simulink model "MPC_HW2_Plant_Simulink"  (R2023b)
settings: Solver=ode4  StartTime=0.0  StopTime=20  FixedStep=1e-3  RelTol=1e-3
values from neighbouring files (symbols this model uses):
  V_ref = 60 /3.6    (= 16.6666666667)    [veh_parameters.m]
undefined symbols (not defined in the file or in its folder): controller_choice, data, init, input, par, Ts
libraries: simulink x6
settings Model: Creator=bshyrokau  LastModifiedBy=india
settings SolverCC: AlgebraicLoopSolver=TrustRegion
settings DataIOCC: SaveOutput=off  SignalLogging=off  DSMLogging=off  SaveTime=off  ReturnWorkspaceOutputs=off
settings OptimizationCC: ReuseModelBlockBuffer=off  LifeSpan=inf
settings DebuggingCC: UnconnectedInputMsg=warning  UnconnectedOutputMsg=warning  UnconnectedLineMsg=warning  AllowSymbolicDim=off  SFUnexpectedBacktrackingDiag=warning  SFNoUnconditionalDefaultTransitionDiag=warning  SFExecutionAtInitializationDiag=none  ArithmeticOperatorsInVariantConditions=warning
settings ModelReferenceCC: EnableRefExpFcnMdlSchedulingChecks=on  PropagateSignalLabelsOutOfModel=off
settings SFSimCC: SimUseLocalCustomCode=off  CustomCodeUndefinedFunction=UseInterfaceOnly
settings RTWCC: RTWUseLocalCustomCode=off  DLArmComputeVersion=19.05
settings CodeAppCC: StateflowObjectComments=on
settings GRTTargetCC: TargetLangStandard=C89/C90 (ANSI)
settings ConfigComp: CovMetricSettings=dw  CovSaveCumulativeToWorkspaceVar=on  CovSaveSingleToWorkspaceVar=on  CovExternalEMLEnable=off
settings SimscapeCC: SimscapeNormalizeSystem=off
settings ConfigurationSet: Description=SimMechanics 2G

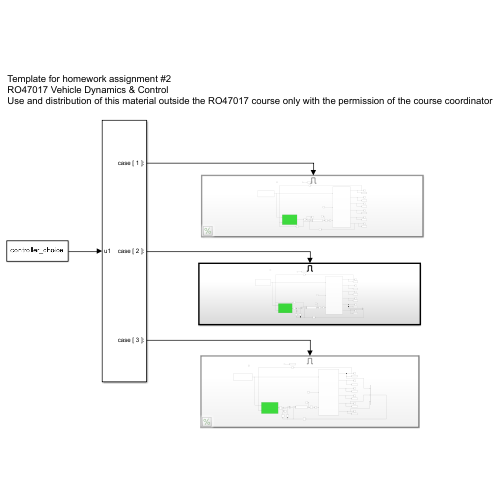
[thumbnail: Simulink's stored preview of the top-level diagram]
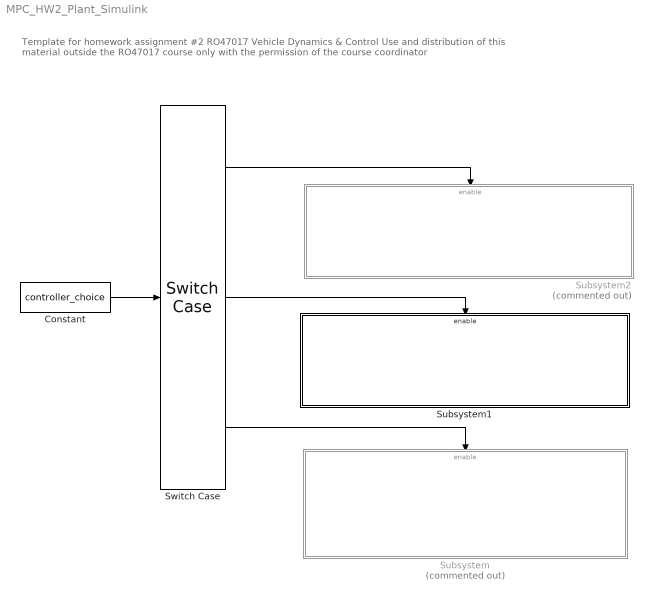
== system MPC_HW2_Plant_Simulink ==
  note: Template for homework assignment #2
      | RO47017 Vehicle Dynamics & Control
      | Use and distribution of this material outside the RO47017 course only with the permission of the course coordinator
  Constant : Constant  Value=controller_choice
  Subsystem : Subsystem  Commented=on
  Subsystem1 : Subsystem
  Subsystem2 : Subsystem  Commented=on
  Switch Case : SwitchCase  CaseConditions={1 2 3}  ShowDefaultCase=off
  wires:
  Switch Case/2 -> Subsystem1/Enable
  Switch Case/3 -> Subsystem/Enable
  Constant/1 -> Switch Case/1
  Switch Case/1 -> Subsystem2/Enable

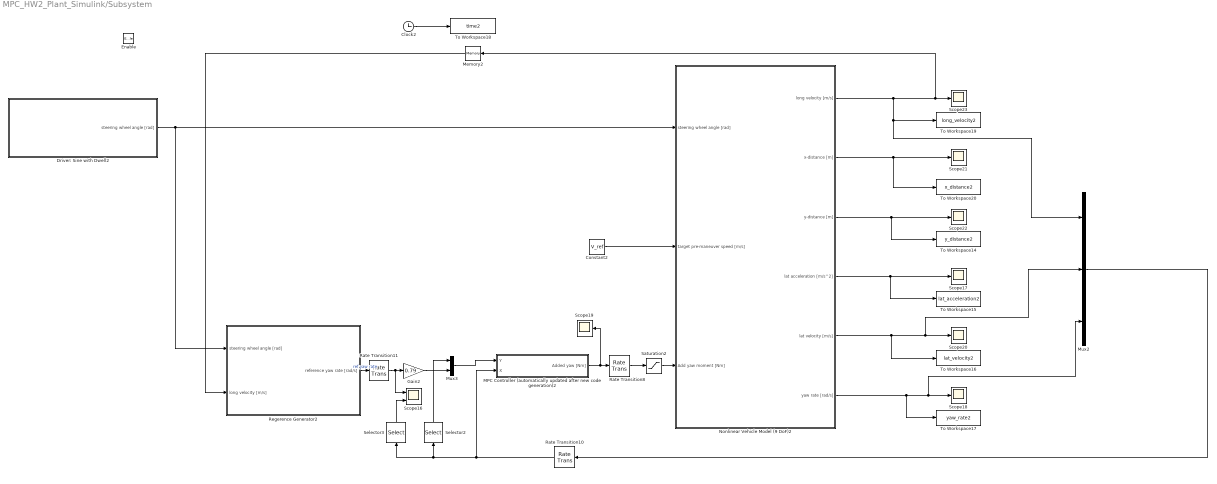
== system MPC_HW2_Plant_Simulink/Subsystem ==
  Enable : EnablePort
  Clock2 : Clock
  Constant2 : Constant  Value=V_ref
  Driver: Sine with Dwell2 : Subsystem
  Gain2 : Gain  Gain=0.79
  MPC Controller (automatically updated after new code generation)2 : Subsystem
  Memory2 : Memory  InitialCondition=V_ref
  Mux2 : Mux  Inputs=3
  Mux3 : Mux  Inputs=2
  Nonlinear Vehicle Model (9 DoF)2 : Subsystem
      mask help: Simulink:masks:GenSFuncDesc_MD
      mask Help: eval('feval(''rtwprivate'',''rtwhelpview'',''rtw_sfcn_block'')');
  Rate Transition10 : RateTransition  InitialCondition=[V_ref 0 0]  OutPortSampleTime=Ts
  Rate Transition11 : RateTransition  OutPortSampleTime=Ts
  Rate Transition8 : RateTransition
  Regerence Generator2 : Subsystem
  Saturation2 : Saturate  UpperLimit=10000  LowerLimit=-10000
  Scope16 : Scope  NumInputPorts=2
  Scope{17..23} (7 alike) : Scope
  Selector2 : Selector  InputPortWidth=3  IndexOptions=Index vector (dialog)  Indices=[1 2]  OutputSizes=1
  Selector3 : Selector  InputPortWidth=3  IndexOptions=Index vector (dialog)  Indices=3  OutputSizes=1
  To Workspace14 : ToWorkspace  VariableName=y_distance2  SampleTime=-1
  To Workspace15 : ToWorkspace  VariableName=lat_acceleration2  SampleTime=-1
  To Workspace16 : ToWorkspace  VariableName=lat_velocity2  SampleTime=-1
  To Workspace17 : ToWorkspace  VariableName=yaw_rate2  SampleTime=-1
  To Workspace18 : ToWorkspace  VariableName=time2  SampleTime=-1
  To Workspace19 : ToWorkspace  VariableName=long_velocity2  SampleTime=-1
  To Workspace20 : ToWorkspace  VariableName=x_distance2  SampleTime=-1
  wires:
  Nonlinear Vehicle Model (9 DoF)2/6(yaw rate [rad/s]) -> Mux2/3, Scope18/1, To Workspace17/1
  Rate Transition10/1 -> Selector3/1, Selector2/1, MPC Controller (automatically updated after new code generation)2/2(X)
  Driver: Sine with Dwell2/1(steering wheel angle [rad]) -> Regerence Generator2/1(steering wheel angle [rad]), Nonlinear Vehicle Model (9 DoF)2/1(steering wheel angle [rad])
  Nonlinear Vehicle Model (9 DoF)2/1(long velocity [m/s]) -> Mux2/1, To Workspace19/1, Memory2/1, Scope23/1
  Nonlinear Vehicle Model (9 DoF)2/5(lat velocity [m/s]) -> To Workspace16/1, Mux2/2, Scope20/1
  Nonlinear Vehicle Model (9 DoF)2/2(x-distance [m]) -> To Workspace20/1, Scope21/1
  Nonlinear Vehicle Model (9 DoF)2/4(lat acceleration [m/s^2]) -> To Workspace15/1, Scope17/1
  MPC Controller (automatically updated after new code generation)2/1(Added yaw [Nm]) -> Scope19/1, Rate Transition8/1
  Mux3/1 -> MPC Controller (automatically updated after new code generation)2/1(Y)
  Mux2/1 -> Rate Transition10/1
  Nonlinear Vehicle Model (9 DoF)2/3(y-distance [m]) -> To Workspace14/1, Scope22/1
  Memory2/1 -> Regerence Generator2/2(long velocity [m/s])
  Selector3/1 -> Scope16/2
  Regerence Generator2/1(reference yaw rate [rad/s]) -> Rate Transition11/1  "ref yaw rate"
  Rate Transition11/1 -> Scope16/1, Gain2/1
  Saturation2/1 -> Nonlinear Vehicle Model (9 DoF)2/3(Add yaw moment [Nm])
  Clock2/1 -> To Workspace18/1
  Rate Transition8/1 -> Saturation2/1
  Constant2/1 -> Nonlinear Vehicle Model (9 DoF)2/2(target pre-maneuver speed [m/s])
  Gain2/1 -> Mux3/2
  Selector2/1 -> Mux3/1

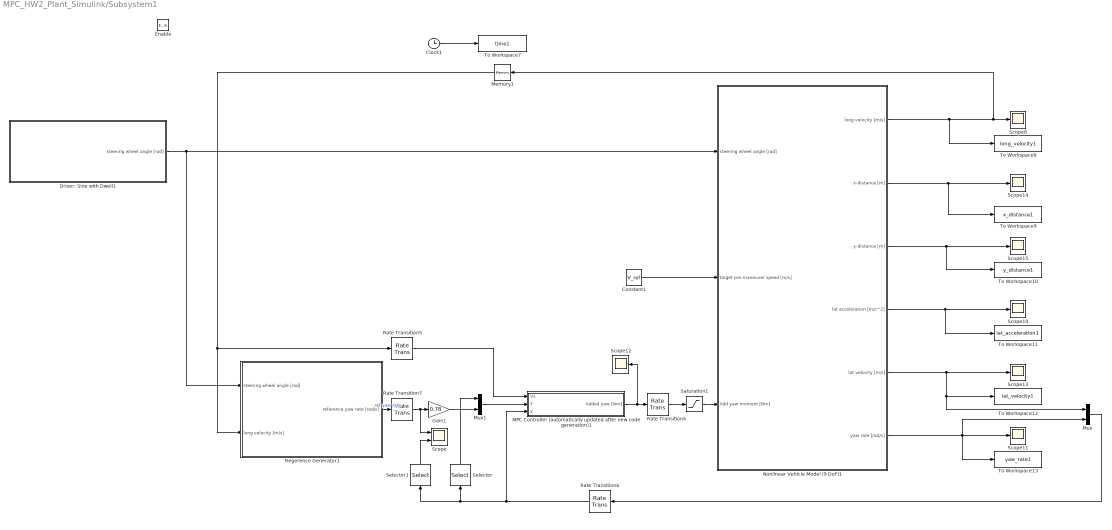
== system MPC_HW2_Plant_Simulink/Subsystem1 ==
  Enable : EnablePort
  Clock1 : Clock
  Constant1 : Constant  Value=V_ref
  Driver: Sine with Dwell1 : Subsystem
  Gain1 : Gain  Gain=0.78
  MPC Controller (automatically updated after new code generation)1 : Subsystem
  Memory1 : Memory  InitialCondition=V_ref
  Mux : Mux  Inputs=2
  Mux1 : Mux  Inputs=2
  Nonlinear Vehicle Model (9 DoF)1 : Subsystem
      mask help: Simulink:masks:GenSFuncDesc_MD
      mask Help: eval('feval(''rtwprivate'',''rtwhelpview'',''rtw_sfcn_block'')');
  Rate Transition4 : RateTransition
  Rate Transition5 : RateTransition  InitialCondition=V_ref  OutPortSampleTime=Ts
  Rate Transition6 : RateTransition  InitialCondition=[0 0]  OutPortSampleTime=Ts
  Rate Transition7 : RateTransition  OutPortSampleTime=Ts
  Regerence Generator1 : Subsystem
  Saturation1 : Saturate  UpperLimit=10000  LowerLimit=-10000
  Scope : Scope  NumInputPorts=2
  Scope{8,10..15} (7 alike) : Scope
  Selector : Selector  InputPortWidth=2  IndexOptions=Index vector (dialog)  Indices=1  OutputSizes=1
  Selector1 : Selector  InputPortWidth=2  IndexOptions=Index vector (dialog)  Indices=2  OutputSizes=1
  To Workspace10 : ToWorkspace  VariableName=y_distance1  SampleTime=-1
  To Workspace11 : ToWorkspace  VariableName=lat_acceleration1  SampleTime=-1
  To Workspace12 : ToWorkspace  VariableName=lat_velocity1  SampleTime=-1
  To Workspace13 : ToWorkspace  VariableName=yaw_rate1  SampleTime=-1
  To Workspace7 : ToWorkspace  VariableName=time1  SampleTime=-1
  To Workspace8 : ToWorkspace  VariableName=long_velocity1  SampleTime=-1
  To Workspace9 : ToWorkspace  VariableName=x_distance1  SampleTime=-1
  wires:
  Rate Transition4/1 -> Saturation1/1
  Nonlinear Vehicle Model (9 DoF)1/3(y-distance [m]) -> To Workspace10/1, Scope15/1
  MPC Controller (automatically updated after new code generation)1/1(Added yaw [Nm]) -> Scope12/1, Rate Transition4/1
  Constant1/1 -> Nonlinear Vehicle Model (9 DoF)1/2(target pre-maneuver speed [m/s])
  Rate Transition6/1 -> Selector1/1, Selector/1, MPC Controller (automatically updated after new code generation)1/3(X)
  Rate Transition5/1 -> MPC Controller (automatically updated after new code generation)1/1(Vx)
  Nonlinear Vehicle Model (9 DoF)1/2(x-distance [m]) -> To Workspace9/1, Scope14/1
  Mux/1 -> Rate Transition6/1
  Saturation1/1 -> Nonlinear Vehicle Model (9 DoF)1/3(Add yaw moment [Nm])
  Nonlinear Vehicle Model (9 DoF)1/1(long velocity [m/s]) -> To Workspace8/1, Memory1/1, Scope8/1
  Regerence Generator1/1(reference yaw rate [rad/s]) -> Rate Transition7/1  "ref yaw rate"
  Memory1/1 -> Regerence Generator1/2(long velocity [m/s]), Rate Transition5/1
  Driver: Sine with Dwell1/1(steering wheel angle [rad]) -> Regerence Generator1/1(steering wheel angle [rad]), Nonlinear Vehicle Model (9 DoF)1/1(steering wheel angle [rad])
  Nonlinear Vehicle Model (9 DoF)1/6(yaw rate [rad/s]) -> Mux/2, Scope11/1, To Workspace13/1
  Clock1/1 -> To Workspace7/1
  Nonlinear Vehicle Model (9 DoF)1/4(lat acceleration [m/s^2]) -> To Workspace11/1, Scope10/1
  Nonlinear Vehicle Model (9 DoF)1/5(lat velocity [m/s]) -> Mux/1, To Workspace12/1, Scope13/1
  Mux1/1 -> MPC Controller (automatically updated after new code generation)1/2(Y)
  Selector1/1 -> Scope/2
  Gain1/1 -> Mux1/2
  Rate Transition7/1 -> Scope/1, Gain1/1
  Selector/1 -> Mux1/1

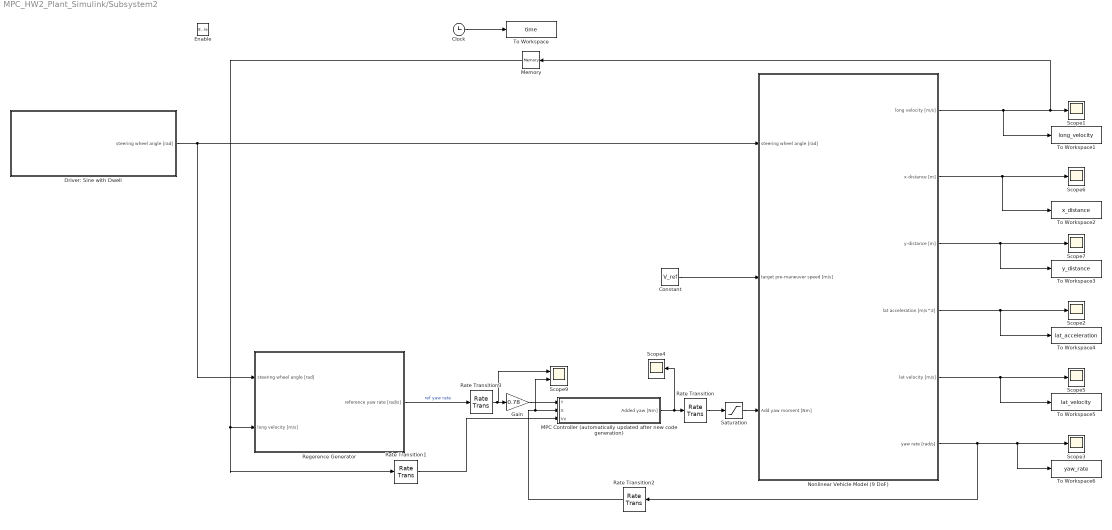
== system MPC_HW2_Plant_Simulink/Subsystem2 ==
  Enable : EnablePort
  Clock : Clock
  Constant : Constant  Value=V_ref
  Driver: Sine with Dwell : Subsystem
  Gain : Gain  Gain=0.78
  MPC Controller (automatically updated after new code generation) : Subsystem
  Memory : Memory  InitialCondition=V_ref
  Nonlinear Vehicle Model (9 DoF) : Subsystem
      mask help: Simulink:masks:GenSFuncDesc_MD
      mask Help: eval('feval(''rtwprivate'',''rtwhelpview'',''rtw_sfcn_block'')');
  Rate Transition : RateTransition
  Rate Transition1 : RateTransition  InitialCondition=V_ref  OutPortSampleTime=Ts
  Rate Transition2 : RateTransition  OutPortSampleTime=Ts
  Rate Transition3 : RateTransition  OutPortSampleTime=Ts
  Regerence Generator : Subsystem
  Saturation : Saturate  UpperLimit=10000  LowerLimit=-10000
  Scope{1..7} (7 alike) : Scope
  Scope9 : Scope  NumInputPorts=2
  To Workspace : ToWorkspace  VariableName=time  SampleTime=-1
  To Workspace1 : ToWorkspace  VariableName=long_velocity  SampleTime=-1
  To Workspace2 : ToWorkspace  VariableName=x_distance  SampleTime=-1
  To Workspace3 : ToWorkspace  VariableName=y_distance  SampleTime=-1
  To Workspace4 : ToWorkspace  VariableName=lat_acceleration  SampleTime=-1
  To Workspace5 : ToWorkspace  VariableName=lat_velocity  SampleTime=-1
  To Workspace6 : ToWorkspace  VariableName=yaw_rate  SampleTime=-1
  wires:
  Driver: Sine with Dwell/1(steering wheel angle [rad]) -> Regerence Generator/1(steering wheel angle [rad]), Nonlinear Vehicle Model (9 DoF)/1(steering wheel angle [rad])
  Nonlinear Vehicle Model (9 DoF)/6(yaw rate [rad/s]) -> Rate Transition2/1, Scope3/1, To Workspace6/1
  Nonlinear Vehicle Model (9 DoF)/3(y-distance [m]) -> To Workspace3/1, Scope7/1
  Nonlinear Vehicle Model (9 DoF)/2(x-distance [m]) -> To Workspace2/1, Scope6/1
  Nonlinear Vehicle Model (9 DoF)/1(long velocity [m/s]) -> To Workspace1/1, Memory/1, Scope1/1
  MPC Controller (automatically updated after new code generation)/1(Added yaw [Nm]) -> Scope4/1, Rate Transition/1
  Gain/1 -> MPC Controller (automatically updated after new code generation)/1(Y)
  Nonlinear Vehicle Model (9 DoF)/5(lat velocity [m/s]) -> To Workspace5/1, Scope5/1
  Rate Transition2/1 -> Scope9/2, MPC Controller (automatically updated after new code generation)/2(X)
  Nonlinear Vehicle Model (9 DoF)/4(lat acceleration [m/s^2]) -> To Workspace4/1, Scope2/1
  Constant/1 -> Nonlinear Vehicle Model (9 DoF)/2(target pre-maneuver speed [m/s])
  Rate Transition3/1 -> Scope9/1, Gain/1
  Memory/1 -> Rate Transition1/1, Regerence Generator/2(long velocity [m/s])
  Clock/1 -> To Workspace/1
  Rate Transition1/1 -> MPC Controller (automatically updated after new code generation)/3(Vx)
  Saturation/1 -> Nonlinear Vehicle Model (9 DoF)/3(Add yaw moment [Nm])
  Regerence Generator/1(reference yaw rate [rad/s]) -> Rate Transition3/1  "ref yaw rate"
  Rate Transition/1 -> Saturation/1

== system MPC_HW2_Plant_Simulink/Subsystem/Driver: Sine with Dwell2 ==
  Constant1 : Constant
  Lookup Table1 : Lookup  InputValues=[0:0.1:3*pi/2 3*pi/2+eps]*0.7  Table=sin([0:0.1:3*pi/2 3*pi/2+eps])  LookUpMeth=Interpolation-Use End Values  SaturateOnIntegerOverflow=off
  Lookup Table2 : Lookup  InputValues=[3*pi/2:0.1:2*pi 2*pi+eps]*0.7  Table=sin([3*pi/2:0.1:2*pi 2*pi+eps])  LookUpMeth=Interpolation-Use End Values  SaturateOnIntegerOverflow=off
  Ramp6 : simulink/Sources/Ramp  slope=pi  start=10  InitialOutput=0
  Ramp7 : simulink/Sources/Ramp  slope=pi  start=10+0.5  InitialOutput=0
  Subtract1 : Sum  Inputs=+++
  amplitude : Gain  Gain=120
  deg2rad : Gain  Gain=pi / 180
  steering wheel angle [rad] : Outport  VectorParamsAs1DForOutWhenUnconnected=off
  wires:
  Ramp6/1 -> Lookup Table1/1
  Ramp7/1 -> Lookup Table2/1
  Lookup Table2/1 -> Subtract1/2
  Lookup Table1/1 -> Subtract1/1
  Constant1/1 -> Subtract1/3
  Subtract1/1 -> amplitude/1
  amplitude/1 -> deg2rad/1
  deg2rad/1 -> steering wheel angle [rad]/1

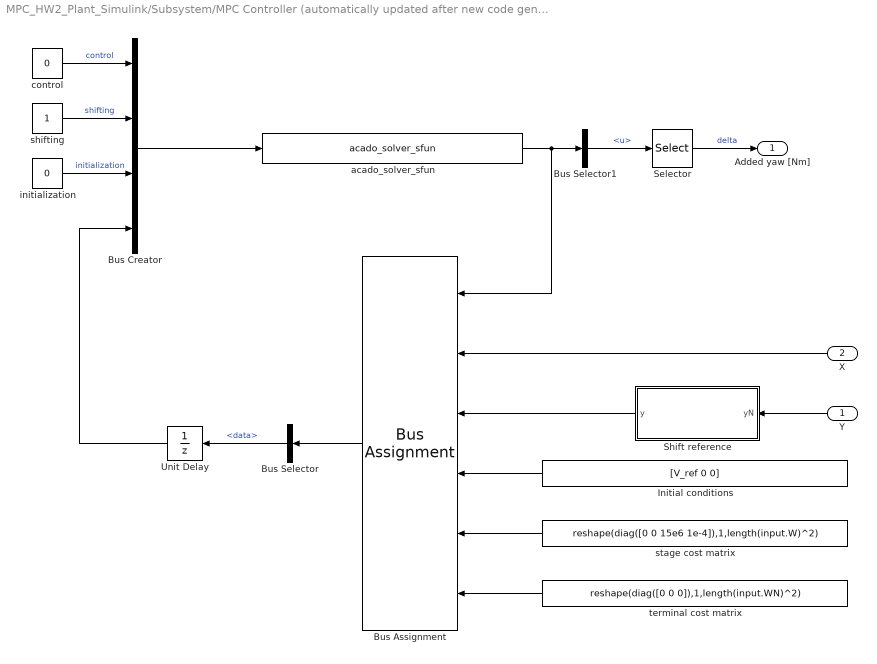
== system MPC_HW2_Plant_Simulink/Subsystem/MPC Controller (automatically updated after new code generation)2 ==
  Y : Inport
  X : Inport  Port=2
  Bus Assignment : BusAssignment  AssignedSignals=data.x0,data.y,data.yN,data.W,data.WN
  Bus Creator : BusCreator  Inputs=4  OutDataTypeStr=Bus: ACADOinput
  Bus Selector : BusSelector  OutputSignals=data
  Bus Selector1 : BusSelector  OutputSignals=data.u
  Initial conditions : Constant  Value=[V_ref 0 0]
  Selector : Selector  InputPortWidth=Np  IndexOptions=Starting index (dialog)  Indices=[1]  OutputSizes=1
  Shift reference : MATLAB Function  TreatAsAtomicUnit=on
  Unit Delay : UnitDelay  InitialCondition=init  SampleTime=Ts  HasFrameUpgradeWarning=on
  acado_solver_sfun : S-Function  FunctionName=acado_solver_sfun  SFunctionDeploymentMode=off  EnableBusSupport=off  mask(Legacy Function){SFunctionSpec=acado_step(ACADOinput u1[1], ACADOoutput y1[1]), ShowSpec=on}
      mask prompts: ShowSpec "Display function specification"
      mask help:
      | This block allows you to call the legacy functions specified by the following Legacy Code Tool definition:
      | def.SFunctionName = 'acado_solver_sfun';
      | def.OutputFcnSpec = 'acado_step(ACADOinput u1[1], ACADOoutput y1[1])';
      | def.StartFcnSpec = 'acado_initialize( void )';
      | def.TerminateFcnSpec = 'acado_cleanup( void )';
      | def.HeaderFiles = {'acado_common.h', 'acado_solver_sfunction.h'};
      | def.SourceFiles = {'acado_solver.c', 'acado_integrator.c', 'acado_auxiliary_functions.c', 'acado_solver_sfunction.c', 'acado_qpoases3_interface.c', 'qpoases3\src\Bounds.c', 'qpoases3\src\Constraints.c', 'qpoases3\src\Indexlist.c', 'qpoases3\src\Matrices.c', 'qpoases3\src\MessageHandling.c', 'qpoases3\src\Options.c', 'qpoases3\src\Flipper.c', 'qpoases3\src\QProblem.c', 'qpoases3\src\QProblemB.c', 'qpoases3\src\Utils.c'};
      mask Help: <p>This block was generated automatically by the Legacy Code Tool. For detailed help on this tool, call<a href="matlab:legacy_code('help')"> legacy_code('help')</a>.</p>
      mask Callback ShowSpec:
      | if strcmp(get_param(gcbh, 'ShowSpec'), 'on')
      |   set_param(gcbh, 'MaskDisplay', sprintf('fprintf(''%s'');', get_param(gcbh, 'SFunctionSpec')));
      | else
      |   set_param(gcbh, 'MaskDisplay', sprintf('fprintf(''%s'');', get_param(gcbh, 'FunctionName')));
      | end
      mask Display: fprintf('acado_step(ACADOinput u1[1], ACADOoutput y1[1])');
  control : Constant  Value=0  OutDataTypeStr=int32
  initialization : Constant  Value=0  OutDataTypeStr=int32
  shifting : Constant  OutDataTypeStr=int32
  stage cost matrix : Constant  Value=reshape(diag([0 0 15e6 1e-4]),1,length(input.W)^2)
  terminal cost matrix : Constant  Value=reshape(diag([0 0 0]),1,length(input.WN)^2)
  Added yaw [Nm] : Outport
  wires:
  control/1 -> Bus Creator/1  "control"
  Bus Selector1/1 -> Selector/1  "<u>"
  initialization/1 -> Bus Creator/3  "initialization"
  acado_solver_sfun/1 -> Bus Selector1/1, Bus Assignment/1
  shifting/1 -> Bus Creator/2  "shifting"
  Bus Assignment/1 -> Bus Selector/1
  terminal cost matrix/1 -> Bus Assignment/6
  Initial conditions/1 -> Bus Assignment/4
  Shift reference/1(y) -> Bus Assignment/3
  stage cost matrix/1 -> Bus Assignment/5
  Bus Selector/1 -> Unit Delay/1  "<data>"
  Unit Delay/1 -> Bus Creator/4
  Bus Creator/1 -> acado_solver_sfun/1
  Selector/1 -> Added yaw [Nm]/1  "delta"
  Y/1 -> Shift reference/1(yN)
  X/1 -> Bus Assignment/2

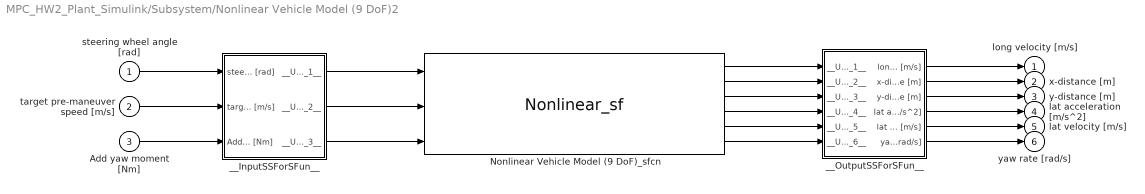
== system MPC_HW2_Plant_Simulink/Subsystem/Nonlinear Vehicle Model (9 DoF)2 ==
  steering wheel angle [rad] : Inport
  target pre-maneuver speed [m/s] : Inport  Port=2
  Add yaw moment [Nm] : Inport  Port=3
  Nonlinear Vehicle Model (9 DoF)_sfcn : S-Function  FunctionName=Nonlinear_sf  SFunctionModules=""  SFunctionDeploymentMode=off  EnableBusSupport=off  mask{rtw_sf_name=Nonlinear_sf, showVar=off}
      mask prompts: rtw_sf_name "Simulink:masks:GenSFuncName_MP"; showVar "Simulink:masks:GenSFuncShowModuleList_MP"
      mask help: Simulink:masks:GenSFuncDesc_MD
      mask init:
      | displist = '';
      | if ~strcmp(get_param(gcb, 'FunctionName'), rtw_sf_name);
      |   set_param(gcb, 'FunctionName', rtw_sf_name);
      | end
      | % Check if we are generating code
      | rtw_mode = false;
      | if strcmpi(get_param(bdroot(gcb),'SimulationStatus'),'Initializing')
      | 	rtw_mode = strcmpi(get_param(bdroot(gcb),'BuildingRTWCode'),'on') && ...
      | 		~strcmpi(get_param(bdroot(gcb),'TargetStyle'),'SimulationTarget');
      | end
      | if showVar || rtw_mode
      | 	if exist('rtwsfunc') == 2 | exist('rtwsfunc') == 6
      | 		tmplist = rtwsfunc(rtw_sf_name,gcb);
      | 		tmplist = DAStudio.message('Simulink:masks:GenSFuncListOfModules_IC', tmplist);
      | 	elseif showVar
      | 		tmplist1 = DAStudio.message('Simulink:masks:GenSFuncListOfModules_IC', '');
      |         tmplist2 = DAStudio.message('Simulink:masks:GenSFuncNotLicensed_IC');
      |         tmplist = [tmplist1 tmplist2];
      |  	end
      | end
      | if showVar
      |   displist = tmplist;
      | end
      settings: CopyFcn=|
      | if ~strcmp(get_param(gcb,'Linkstatus'),'none') && ...
      | ~strcmp(get_param(gcb,'Linkstatus'),'implicit')
      |   set_param(gcb,'LinkStatus','none');
      | end
      mask Help: eval('feval(''rtwprivate'',''rtwhelpview'',''rtw_sfcn_block'')');
      mask Display:
      | port_label('input',1,'steering wheel angle [rad]');
      | port_label('input',2,'target pre-maneuver speed [m/s]');
      | port_label('input',3,'Add yaw moment [Nm]');
      | port_label('output',1,'long velocity [m/s]');
      | port_label('output',2,'x-distance [m]');
      | port_label('output',3,'y-distance [m]');
      | port_label('output',4,'lat acceleration [m/s^2]');
      | port_label('output',5,'lat velocity [m/s]');
      | port_label('output',6,'yaw rate [rad/s]');
  __InputSSForSFun__ : Subsystem
  __OutputSSForSFun__ : Subsystem
  long velocity [m/s] : Outport  VectorParamsAs1DForOutWhenUnconnected=off
  x-distance [m] : Outport  Port=2  VectorParamsAs1DForOutWhenUnconnected=off
  y-distance [m] : Outport  Port=3  VectorParamsAs1DForOutWhenUnconnected=off
  lat acceleration [m/s^2] : Outport  Port=4  VectorParamsAs1DForOutWhenUnconnected=off
  lat velocity [m/s] : Outport  Port=5  VectorParamsAs1DForOutWhenUnconnected=off
  yaw rate [rad/s] : Outport  Port=6  VectorParamsAs1DForOutWhenUnconnected=off
  wires:
  steering wheel angle [rad]/1 -> __InputSSForSFun__/1(steering wheel angle [rad])
  target pre-maneuver speed [m/s]/1 -> __InputSSForSFun__/2(target pre-maneuver speed [m/s])
  __InputSSForSFun__/1(__UniqueOutportName__1__) -> Nonlinear Vehicle Model (9 DoF)_sfcn/1
  __InputSSForSFun__/3(__UniqueOutportName__3__) -> Nonlinear Vehicle Model (9 DoF)_sfcn/3
  Nonlinear Vehicle Model (9 DoF)_sfcn/1 -> __OutputSSForSFun__/1(__UniqueInportName__1__)
  Nonlinear Vehicle Model (9 DoF)_sfcn/2 -> __OutputSSForSFun__/2(__UniqueInportName__2__)
  Nonlinear Vehicle Model (9 DoF)_sfcn/3 -> __OutputSSForSFun__/3(__UniqueInportName__3__)
  Nonlinear Vehicle Model (9 DoF)_sfcn/4 -> __OutputSSForSFun__/4(__UniqueInportName__4__)
  Nonlinear Vehicle Model (9 DoF)_sfcn/5 -> __OutputSSForSFun__/5(__UniqueInportName__5__)
  Nonlinear Vehicle Model (9 DoF)_sfcn/6 -> __OutputSSForSFun__/6(__UniqueInportName__6__)
  __OutputSSForSFun__/1(long velocity [m/s]) -> long velocity [m/s]/1
  __OutputSSForSFun__/2(x-distance [m]) -> x-distance [m]/1
  __OutputSSForSFun__/3(y-distance [m]) -> y-distance [m]/1
  __OutputSSForSFun__/4(lat acceleration [m/s^2]) -> lat acceleration [m/s^2]/1
  __OutputSSForSFun__/5(lat velocity [m/s]) -> lat velocity [m/s]/1
  __OutputSSForSFun__/6(yaw rate [rad/s]) -> yaw rate [rad/s]/1
  __InputSSForSFun__/2(__UniqueOutportName__2__) -> Nonlinear Vehicle Model (9 DoF)_sfcn/2
  Add yaw moment [Nm]/1 -> __InputSSForSFun__/3(Add yaw moment [Nm])

== system MPC_HW2_Plant_Simulink/Subsystem/Regerence Generator2 ==
  note: yawr_ref
  note: nonlinear response
  note: delta
  note: u
  steering wheel angle [rad] : Inport
  long velocity [m/s] : Inport  Port=2
  MATLAB Function : MATLAB Function  TreatAsAtomicUnit=on
  MATLAB Function1 : MATLAB Function  TreatAsAtomicUnit=on
  Transfer Fcn : TransferFcn  Numerator=[par.wn^2*par.tau par.wn^2]  Denominator=[1 2*par.kseta*par.wn par.wn^2]
  steering ratio : Gain  Gain=1/ par.i_steer
  reference yaw rate [rad/s] : Outport  VectorParamsAs1DForOutWhenUnconnected=off
  wires:
  steering wheel angle [rad]/1 -> steering ratio/1
  steering ratio/1 -> MATLAB Function/1(delta)
  long velocity [m/s]/1 -> MATLAB Function1/2(u), MATLAB Function/2(u)
  MATLAB Function/1(yawr_ss) -> MATLAB Function1/1(yawr_ss)
  MATLAB Function1/1(yawr_sat) -> Transfer Fcn/1
  Transfer Fcn/1 -> reference yaw rate [rad/s]/1

== system MPC_HW2_Plant_Simulink/Subsystem1/Driver: Sine with Dwell1 ==
  Constant1 : Constant
  Lookup Table1 : Lookup  InputValues=[0:0.1:3*pi/2 3*pi/2+eps]*0.7  Table=sin([0:0.1:3*pi/2 3*pi/2+eps])  LookUpMeth=Interpolation-Use End Values  SaturateOnIntegerOverflow=off
  Lookup Table2 : Lookup  InputValues=[3*pi/2:0.1:2*pi 2*pi+eps]*0.7  Table=sin([3*pi/2:0.1:2*pi 2*pi+eps])  LookUpMeth=Interpolation-Use End Values  SaturateOnIntegerOverflow=off
  Ramp6 : simulink/Sources/Ramp  slope=pi  start=10  InitialOutput=0
  Ramp7 : simulink/Sources/Ramp  slope=pi  start=10+0.5  InitialOutput=0
  Subtract1 : Sum  Inputs=+++
  amplitude : Gain  Gain=120
  deg2rad : Gain  Gain=pi / 180
  steering wheel angle [rad] : Outport  VectorParamsAs1DForOutWhenUnconnected=off
  wires:
  Ramp6/1 -> Lookup Table1/1
  Ramp7/1 -> Lookup Table2/1
  Lookup Table2/1 -> Subtract1/2
  Lookup Table1/1 -> Subtract1/1
  Constant1/1 -> Subtract1/3
  Subtract1/1 -> amplitude/1
  amplitude/1 -> deg2rad/1
  deg2rad/1 -> steering wheel angle [rad]/1

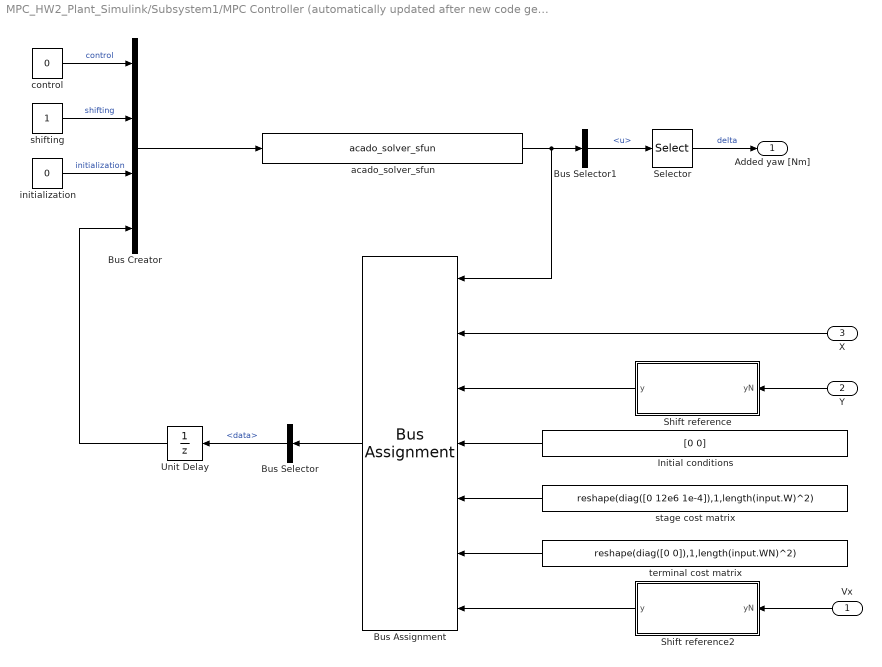
== system MPC_HW2_Plant_Simulink/Subsystem1/MPC Controller (automatically updated after new code generation)1 ==
  Vx : Inport
  Y : Inport  Port=2
  X : Inport  Port=3
  Bus Assignment : BusAssignment  AssignedSignals=data.x0,data.y,data.yN,data.W,data.WN,data.od
  Bus Creator : BusCreator  Inputs=4  OutDataTypeStr=Bus: ACADOinput
  Bus Selector : BusSelector  OutputSignals=data
  Bus Selector1 : BusSelector  OutputSignals=data.u
  Initial conditions : Constant  Value=[0 0]
  Selector : Selector  InputPortWidth=Np  IndexOptions=Starting index (dialog)  Indices=[1]  OutputSizes=1
  Shift reference : MATLAB Function  TreatAsAtomicUnit=on
  Shift reference2 : MATLAB Function  TreatAsAtomicUnit=on
  Unit Delay : UnitDelay  InitialCondition=init  SampleTime=Ts  HasFrameUpgradeWarning=on
  acado_solver_sfun : S-Function  FunctionName=acado_solver_sfun  SFunctionDeploymentMode=off  EnableBusSupport=off  mask(Legacy Function){SFunctionSpec=acado_step(ACADOinput u1[1], ACADOoutput y1[1]), ShowSpec=on}
      mask prompts: ShowSpec "Display function specification"
      mask help:
      | This block allows you to call the legacy functions specified by the following Legacy Code Tool definition:
      | def.SFunctionName = 'acado_solver_sfun';
      | def.OutputFcnSpec = 'acado_step(ACADOinput u1[1], ACADOoutput y1[1])';
      | def.StartFcnSpec = 'acado_initialize( void )';
      | def.TerminateFcnSpec = 'acado_cleanup( void )';
      | def.HeaderFiles = {'acado_common.h', 'acado_solver_sfunction.h'};
      | def.SourceFiles = {'acado_solver.c', 'acado_integrator.c', 'acado_auxiliary_functions.c', 'acado_solver_sfunction.c', 'acado_qpoases3_interface.c', 'qpoases3\src\Bounds.c', 'qpoases3\src\Constraints.c', 'qpoases3\src\Indexlist.c', 'qpoases3\src\Matrices.c', 'qpoases3\src\MessageHandling.c', 'qpoases3\src\Options.c', 'qpoases3\src\Flipper.c', 'qpoases3\src\QProblem.c', 'qpoases3\src\QProblemB.c', 'qpoases3\src\Utils.c'};
      mask Help: <p>This block was generated automatically by the Legacy Code Tool. For detailed help on this tool, call<a href="matlab:legacy_code('help')"> legacy_code('help')</a>.</p>
      mask Callback ShowSpec:
      | if strcmp(get_param(gcbh, 'ShowSpec'), 'on')
      |   set_param(gcbh, 'MaskDisplay', sprintf('fprintf(''%s'');', get_param(gcbh, 'SFunctionSpec')));
      | else
      |   set_param(gcbh, 'MaskDisplay', sprintf('fprintf(''%s'');', get_param(gcbh, 'FunctionName')));
      | end
      mask Display: fprintf('acado_step(ACADOinput u1[1], ACADOoutput y1[1])');
  control : Constant  Value=0  OutDataTypeStr=int32
  initialization : Constant  Value=0  OutDataTypeStr=int32
  shifting : Constant  OutDataTypeStr=int32
  stage cost matrix : Constant  Value=reshape(diag([0 12e6 1e-4]),1,length(input.W)^2)
  terminal cost matrix : Constant  Value=reshape(diag([0 0]),1,length(input.WN)^2)
  Added yaw [Nm] : Outport
  wires:
  control/1 -> Bus Creator/1  "control"
  Bus Selector1/1 -> Selector/1  "<u>"
  initialization/1 -> Bus Creator/3  "initialization"
  acado_solver_sfun/1 -> Bus Selector1/1, Bus Assignment/1
  shifting/1 -> Bus Creator/2  "shifting"
  Bus Assignment/1 -> Bus Selector/1
  terminal cost matrix/1 -> Bus Assignment/6
  Initial conditions/1 -> Bus Assignment/4
  Shift reference/1(y) -> Bus Assignment/3
  stage cost matrix/1 -> Bus Assignment/5
  Bus Selector/1 -> Unit Delay/1  "<data>"
  Unit Delay/1 -> Bus Creator/4
  Bus Creator/1 -> acado_solver_sfun/1
  Selector/1 -> Added yaw [Nm]/1  "delta"
  Y/1 -> Shift reference/1(yN)
  X/1 -> Bus Assignment/2
  Shift reference2/1(y) -> Bus Assignment/7
  Vx/1 -> Shift reference2/1(yN)

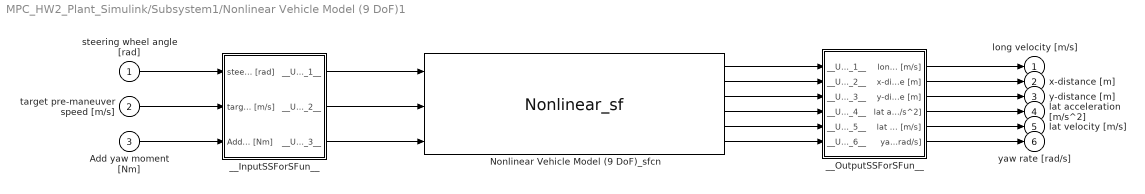
== system MPC_HW2_Plant_Simulink/Subsystem1/Nonlinear Vehicle Model (9 DoF)1 ==
  steering wheel angle [rad] : Inport
  target pre-maneuver speed [m/s] : Inport  Port=2
  Add yaw moment [Nm] : Inport  Port=3
  Nonlinear Vehicle Model (9 DoF)_sfcn : S-Function  FunctionName=Nonlinear_sf  SFunctionModules=""  SFunctionDeploymentMode=off  EnableBusSupport=off  mask{rtw_sf_name=Nonlinear_sf, showVar=off}
      mask prompts: rtw_sf_name "Simulink:masks:GenSFuncName_MP"; showVar "Simulink:masks:GenSFuncShowModuleList_MP"
      mask help: Simulink:masks:GenSFuncDesc_MD
      mask init: same as MPC_HW2_Plant_Simulink/Subsystem/Nonlinear Vehicle Model (9 DoF)2/Nonlinear Vehicle Model (9 DoF)_sfcn
      settings: CopyFcn=|
      | if ~strcmp(get_param(gcb,'Linkstatus'),'none') && ...
      | ~strcmp(get_param(gcb,'Linkstatus'),'implicit')
      |   set_param(gcb,'LinkStatus','none');
      | end
      mask Help: eval('feval(''rtwprivate'',''rtwhelpview'',''rtw_sfcn_block'')');
      mask Display:
      | port_label('input',1,'steering wheel angle [rad]');
      | port_label('input',2,'target pre-maneuver speed [m/s]');
      | port_label('input',3,'Add yaw moment [Nm]');
      | port_label('output',1,'long velocity [m/s]');
      | port_label('output',2,'x-distance [m]');
      | port_label('output',3,'y-distance [m]');
      | port_label('output',4,'lat acceleration [m/s^2]');
      | port_label('output',5,'lat velocity [m/s]');
      | port_label('output',6,'yaw rate [rad/s]');
  __InputSSForSFun__ : Subsystem
  __OutputSSForSFun__ : Subsystem
  long velocity [m/s] : Outport  VectorParamsAs1DForOutWhenUnconnected=off
  x-distance [m] : Outport  Port=2  VectorParamsAs1DForOutWhenUnconnected=off
  y-distance [m] : Outport  Port=3  VectorParamsAs1DForOutWhenUnconnected=off
  lat acceleration [m/s^2] : Outport  Port=4  VectorParamsAs1DForOutWhenUnconnected=off
  lat velocity [m/s] : Outport  Port=5  VectorParamsAs1DForOutWhenUnconnected=off
  yaw rate [rad/s] : Outport  Port=6  VectorParamsAs1DForOutWhenUnconnected=off
  wires:
  steering wheel angle [rad]/1 -> __InputSSForSFun__/1(steering wheel angle [rad])
  target pre-maneuver speed [m/s]/1 -> __InputSSForSFun__/2(target pre-maneuver speed [m/s])
  __InputSSForSFun__/1(__UniqueOutportName__1__) -> Nonlinear Vehicle Model (9 DoF)_sfcn/1
  __InputSSForSFun__/3(__UniqueOutportName__3__) -> Nonlinear Vehicle Model (9 DoF)_sfcn/3
  Nonlinear Vehicle Model (9 DoF)_sfcn/1 -> __OutputSSForSFun__/1(__UniqueInportName__1__)
  Nonlinear Vehicle Model (9 DoF)_sfcn/2 -> __OutputSSForSFun__/2(__UniqueInportName__2__)
  Nonlinear Vehicle Model (9 DoF)_sfcn/3 -> __OutputSSForSFun__/3(__UniqueInportName__3__)
  Nonlinear Vehicle Model (9 DoF)_sfcn/4 -> __OutputSSForSFun__/4(__UniqueInportName__4__)
  Nonlinear Vehicle Model (9 DoF)_sfcn/5 -> __OutputSSForSFun__/5(__UniqueInportName__5__)
  Nonlinear Vehicle Model (9 DoF)_sfcn/6 -> __OutputSSForSFun__/6(__UniqueInportName__6__)
  __OutputSSForSFun__/1(long velocity [m/s]) -> long velocity [m/s]/1
  __OutputSSForSFun__/2(x-distance [m]) -> x-distance [m]/1
  __OutputSSForSFun__/3(y-distance [m]) -> y-distance [m]/1
  __OutputSSForSFun__/4(lat acceleration [m/s^2]) -> lat acceleration [m/s^2]/1
  __OutputSSForSFun__/5(lat velocity [m/s]) -> lat velocity [m/s]/1
  __OutputSSForSFun__/6(yaw rate [rad/s]) -> yaw rate [rad/s]/1
  __InputSSForSFun__/2(__UniqueOutportName__2__) -> Nonlinear Vehicle Model (9 DoF)_sfcn/2
  Add yaw moment [Nm]/1 -> __InputSSForSFun__/3(Add yaw moment [Nm])

== system MPC_HW2_Plant_Simulink/Subsystem1/Regerence Generator1 ==
  note: yawr_ref
  note: nonlinear response
  note: delta
  note: u
  steering wheel angle [rad] : Inport
  long velocity [m/s] : Inport  Port=2
  MATLAB Function : MATLAB Function  TreatAsAtomicUnit=on
  MATLAB Function1 : MATLAB Function  TreatAsAtomicUnit=on
  Transfer Fcn : TransferFcn  Numerator=[par.wn^2*par.tau par.wn^2]  Denominator=[1 2*par.kseta*par.wn par.wn^2]
  steering ratio : Gain  Gain=1/ par.i_steer
  reference yaw rate [rad/s] : Outport  VectorParamsAs1DForOutWhenUnconnected=off
  wires:
  steering wheel angle [rad]/1 -> steering ratio/1
  steering ratio/1 -> MATLAB Function/1(delta)
  long velocity [m/s]/1 -> MATLAB Function1/2(u), MATLAB Function/2(u)
  MATLAB Function/1(yawr_ss) -> MATLAB Function1/1(yawr_ss)
  MATLAB Function1/1(yawr_sat) -> Transfer Fcn/1
  Transfer Fcn/1 -> reference yaw rate [rad/s]/1

== system MPC_HW2_Plant_Simulink/Subsystem2/Driver: Sine with Dwell ==
  Constant1 : Constant
  Lookup Table1 : Lookup  InputValues=[0:0.1:3*pi/2 3*pi/2+eps]*0.7  Table=sin([0:0.1:3*pi/2 3*pi/2+eps])  LookUpMeth=Interpolation-Use End Values  SaturateOnIntegerOverflow=off
  Lookup Table2 : Lookup  InputValues=[3*pi/2:0.1:2*pi 2*pi+eps]*0.7  Table=sin([3*pi/2:0.1:2*pi 2*pi+eps])  LookUpMeth=Interpolation-Use End Values  SaturateOnIntegerOverflow=off
  Ramp6 : simulink/Sources/Ramp  slope=pi  start=10  InitialOutput=0
  Ramp7 : simulink/Sources/Ramp  slope=pi  start=10+0.5  InitialOutput=0
  Subtract1 : Sum  Inputs=+++
  amplitude : Gain  Gain=120
  deg2rad : Gain  Gain=pi / 180
  steering wheel angle [rad] : Outport  VectorParamsAs1DForOutWhenUnconnected=off
  wires:
  Ramp6/1 -> Lookup Table1/1
  Ramp7/1 -> Lookup Table2/1
  Lookup Table2/1 -> Subtract1/2
  Lookup Table1/1 -> Subtract1/1
  Constant1/1 -> Subtract1/3
  Subtract1/1 -> amplitude/1
  amplitude/1 -> deg2rad/1
  deg2rad/1 -> steering wheel angle [rad]/1

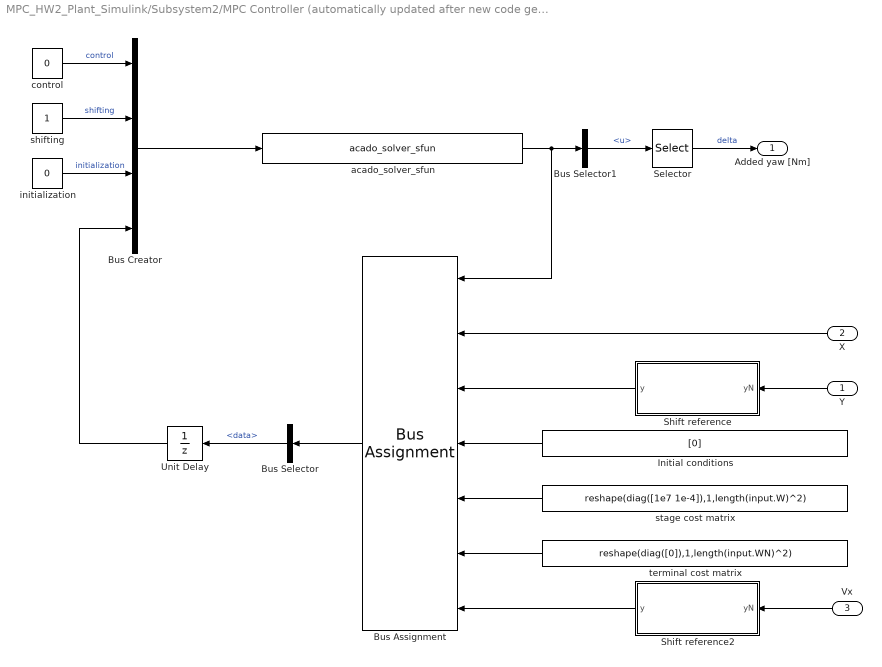
== system MPC_HW2_Plant_Simulink/Subsystem2/MPC Controller (automatically updated after new code generation) ==
  Y : Inport
  X : Inport  Port=2
  Vx : Inport  Port=3
  Bus Assignment : BusAssignment  AssignedSignals=data.x0,data.y,data.yN,data.W,data.WN,data.od
  Bus Creator : BusCreator  Inputs=4  OutDataTypeStr=Bus: ACADOinput
  Bus Selector : BusSelector  OutputSignals=data
  Bus Selector1 : BusSelector  OutputSignals=data.u
  Initial conditions : Constant  Value=[0]
  Selector : Selector  InputPortWidth=Np  IndexOptions=Starting index (dialog)  Indices=[1]  OutputSizes=1
  Shift reference : MATLAB Function  TreatAsAtomicUnit=on
  Shift reference2 : MATLAB Function  TreatAsAtomicUnit=on
  Unit Delay : UnitDelay  InitialCondition=init  SampleTime=Ts  HasFrameUpgradeWarning=on
  acado_solver_sfun : S-Function  FunctionName=acado_solver_sfun  SFunctionDeploymentMode=off  EnableBusSupport=off  mask(Legacy Function){SFunctionSpec=acado_step(ACADOinput u1[1], ACADOoutput y1[1]), ShowSpec=on}
      mask prompts: ShowSpec "Display function specification"
      mask help:
      | This block allows you to call the legacy functions specified by the following Legacy Code Tool definition:
      | def.SFunctionName = 'acado_solver_sfun';
      | def.OutputFcnSpec = 'acado_step(ACADOinput u1[1], ACADOoutput y1[1])';
      | def.StartFcnSpec = 'acado_initialize( void )';
      | def.TerminateFcnSpec = 'acado_cleanup( void )';
      | def.HeaderFiles = {'acado_common.h', 'acado_solver_sfunction.h'};
      | def.SourceFiles = {'acado_solver.c', 'acado_integrator.c', 'acado_auxiliary_functions.c', 'acado_solver_sfunction.c', 'acado_qpoases3_interface.c', 'qpoases3\src\Bounds.c', 'qpoases3\src\Constraints.c', 'qpoases3\src\Indexlist.c', 'qpoases3\src\Matrices.c', 'qpoases3\src\MessageHandling.c', 'qpoases3\src\Options.c', 'qpoases3\src\Flipper.c', 'qpoases3\src\QProblem.c', 'qpoases3\src\QProblemB.c', 'qpoases3\src\Utils.c'};
      mask Help: <p>This block was generated automatically by the Legacy Code Tool. For detailed help on this tool, call<a href="matlab:legacy_code('help')"> legacy_code('help')</a>.</p>
      mask Callback ShowSpec:
      | if strcmp(get_param(gcbh, 'ShowSpec'), 'on')
      |   set_param(gcbh, 'MaskDisplay', sprintf('fprintf(''%s'');', get_param(gcbh, 'SFunctionSpec')));
      | else
      |   set_param(gcbh, 'MaskDisplay', sprintf('fprintf(''%s'');', get_param(gcbh, 'FunctionName')));
      | end
      mask Display: fprintf('acado_step(ACADOinput u1[1], ACADOoutput y1[1])');
  control : Constant  Value=0  OutDataTypeStr=int32
  initialization : Constant  Value=0  OutDataTypeStr=int32
  shifting : Constant  OutDataTypeStr=int32
  stage cost matrix : Constant  Value=reshape(diag([1e7 1e-4]),1,length(input.W)^2)
  terminal cost matrix : Constant  Value=reshape(diag([0]),1,length(input.WN)^2)
  Added yaw [Nm] : Outport
  wires:
  control/1 -> Bus Creator/1  "control"
  Bus Selector1/1 -> Selector/1  "<u>"
  initialization/1 -> Bus Creator/3  "initialization"
  acado_solver_sfun/1 -> Bus Selector1/1, Bus Assignment/1
  shifting/1 -> Bus Creator/2  "shifting"
  Bus Assignment/1 -> Bus Selector/1
  terminal cost matrix/1 -> Bus Assignment/6
  Initial conditions/1 -> Bus Assignment/4
  Shift reference/1(y) -> Bus Assignment/3
  stage cost matrix/1 -> Bus Assignment/5
  Bus Selector/1 -> Unit Delay/1  "<data>"
  Unit Delay/1 -> Bus Creator/4
  Bus Creator/1 -> acado_solver_sfun/1
  Selector/1 -> Added yaw [Nm]/1  "delta"
  Y/1 -> Shift reference/1(yN)
  X/1 -> Bus Assignment/2
  Shift reference2/1(y) -> Bus Assignment/7
  Vx/1 -> Shift reference2/1(yN)

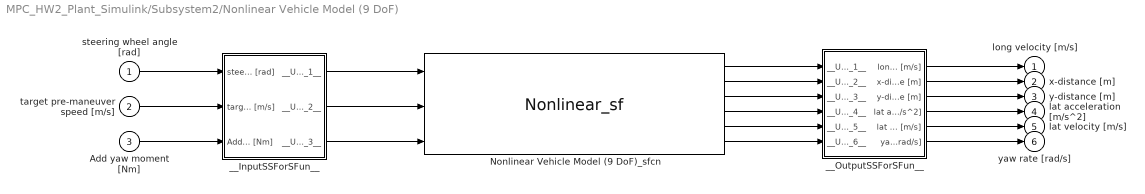
== system MPC_HW2_Plant_Simulink/Subsystem2/Nonlinear Vehicle Model (9 DoF) ==
  steering wheel angle [rad] : Inport
  target pre-maneuver speed [m/s] : Inport  Port=2
  Add yaw moment [Nm] : Inport  Port=3
  Nonlinear Vehicle Model (9 DoF)_sfcn : S-Function  FunctionName=Nonlinear_sf  SFunctionModules=""  SFunctionDeploymentMode=off  EnableBusSupport=off  mask{rtw_sf_name=Nonlinear_sf, showVar=off}
      mask prompts: rtw_sf_name "Simulink:masks:GenSFuncName_MP"; showVar "Simulink:masks:GenSFuncShowModuleList_MP"
      mask help: Simulink:masks:GenSFuncDesc_MD
      mask init: same as MPC_HW2_Plant_Simulink/Subsystem/Nonlinear Vehicle Model (9 DoF)2/Nonlinear Vehicle Model (9 DoF)_sfcn
      settings: CopyFcn=|
      | if ~strcmp(get_param(gcb,'Linkstatus'),'none') && ...
      | ~strcmp(get_param(gcb,'Linkstatus'),'implicit')
      |   set_param(gcb,'LinkStatus','none');
      | end
      mask Help: eval('feval(''rtwprivate'',''rtwhelpview'',''rtw_sfcn_block'')');
      mask Display:
      | port_label('input',1,'steering wheel angle [rad]');
      | port_label('input',2,'target pre-maneuver speed [m/s]');
      | port_label('input',3,'Add yaw moment [Nm]');
      | port_label('output',1,'long velocity [m/s]');
      | port_label('output',2,'x-distance [m]');
      | port_label('output',3,'y-distance [m]');
      | port_label('output',4,'lat acceleration [m/s^2]');
      | port_label('output',5,'lat velocity [m/s]');
      | port_label('output',6,'yaw rate [rad/s]');
  __InputSSForSFun__ : Subsystem
  __OutputSSForSFun__ : Subsystem
  long velocity [m/s] : Outport  VectorParamsAs1DForOutWhenUnconnected=off
  x-distance [m] : Outport  Port=2  VectorParamsAs1DForOutWhenUnconnected=off
  y-distance [m] : Outport  Port=3  VectorParamsAs1DForOutWhenUnconnected=off
  lat acceleration [m/s^2] : Outport  Port=4  VectorParamsAs1DForOutWhenUnconnected=off
  lat velocity [m/s] : Outport  Port=5  VectorParamsAs1DForOutWhenUnconnected=off
  yaw rate [rad/s] : Outport  Port=6  VectorParamsAs1DForOutWhenUnconnected=off
  wires:
  steering wheel angle [rad]/1 -> __InputSSForSFun__/1(steering wheel angle [rad])
  target pre-maneuver speed [m/s]/1 -> __InputSSForSFun__/2(target pre-maneuver speed [m/s])
  __InputSSForSFun__/1(__UniqueOutportName__1__) -> Nonlinear Vehicle Model (9 DoF)_sfcn/1
  __InputSSForSFun__/3(__UniqueOutportName__3__) -> Nonlinear Vehicle Model (9 DoF)_sfcn/3
  Nonlinear Vehicle Model (9 DoF)_sfcn/1 -> __OutputSSForSFun__/1(__UniqueInportName__1__)
  Nonlinear Vehicle Model (9 DoF)_sfcn/2 -> __OutputSSForSFun__/2(__UniqueInportName__2__)
  Nonlinear Vehicle Model (9 DoF)_sfcn/3 -> __OutputSSForSFun__/3(__UniqueInportName__3__)
  Nonlinear Vehicle Model (9 DoF)_sfcn/4 -> __OutputSSForSFun__/4(__UniqueInportName__4__)
  Nonlinear Vehicle Model (9 DoF)_sfcn/5 -> __OutputSSForSFun__/5(__UniqueInportName__5__)
  Nonlinear Vehicle Model (9 DoF)_sfcn/6 -> __OutputSSForSFun__/6(__UniqueInportName__6__)
  __OutputSSForSFun__/1(long velocity [m/s]) -> long velocity [m/s]/1
  __OutputSSForSFun__/2(x-distance [m]) -> x-distance [m]/1
  __OutputSSForSFun__/3(y-distance [m]) -> y-distance [m]/1
  __OutputSSForSFun__/4(lat acceleration [m/s^2]) -> lat acceleration [m/s^2]/1
  __OutputSSForSFun__/5(lat velocity [m/s]) -> lat velocity [m/s]/1
  __OutputSSForSFun__/6(yaw rate [rad/s]) -> yaw rate [rad/s]/1
  __InputSSForSFun__/2(__UniqueOutportName__2__) -> Nonlinear Vehicle Model (9 DoF)_sfcn/2
  Add yaw moment [Nm]/1 -> __InputSSForSFun__/3(Add yaw moment [Nm])

== system MPC_HW2_Plant_Simulink/Subsystem2/Regerence Generator ==
  note: yawr_ref
  note: nonlinear response
  note: delta
  note: u
  steering wheel angle [rad] : Inport
  long velocity [m/s] : Inport  Port=2
  MATLAB Function : MATLAB Function  TreatAsAtomicUnit=on
  MATLAB Function1 : MATLAB Function  TreatAsAtomicUnit=on
  Transfer Fcn : TransferFcn  Numerator=[par.wn^2*par.tau par.wn^2]  Denominator=[1 2*par.kseta*par.wn par.wn^2]
  steering ratio : Gain  Gain=1/ par.i_steer
  reference yaw rate [rad/s] : Outport  VectorParamsAs1DForOutWhenUnconnected=off
  wires:
  steering wheel angle [rad]/1 -> steering ratio/1
  steering ratio/1 -> MATLAB Function/1(delta)
  long velocity [m/s]/1 -> MATLAB Function1/2(u), MATLAB Function/2(u)
  MATLAB Function/1(yawr_ss) -> MATLAB Function1/1(yawr_ss)
  MATLAB Function1/1(yawr_sat) -> Transfer Fcn/1
  Transfer Fcn/1 -> reference yaw rate [rad/s]/1

== system MPC_HW2_Plant_Simulink/Subsystem/Nonlinear Vehicle Model (9 DoF)2/__InputSSForSFun__ ==
  steering wheel angle [rad] : Inport
  target pre-maneuver speed [m/s] : Inport  Port=2
  Add yaw moment [Nm] : Inport  Port=3
  __UniqueOutportName__1__ : Outport
  __UniqueOutportName__2__ : Outport  Port=2
  __UniqueOutportName__3__ : Outport  Port=3
  wires:
  steering wheel angle [rad]/1 -> __UniqueOutportName__1__/1
  target pre-maneuver speed [m/s]/1 -> __UniqueOutportName__2__/1
  Add yaw moment [Nm]/1 -> __UniqueOutportName__3__/1

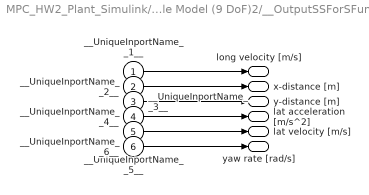
== system MPC_HW2_Plant_Simulink/Subsystem/Nonlinear Vehicle Model (9 DoF)2/__OutputSSForSFun__ ==
  __UniqueInportName__1__ : Inport
  __UniqueInportName__2__ : Inport  Port=2
  __UniqueInportName__3__ : Inport  Port=3
  __UniqueInportName__4__ : Inport  Port=4
  __UniqueInportName__5__ : Inport  Port=5
  __UniqueInportName__6__ : Inport  Port=6
  long velocity [m/s] : Outport  VectorParamsAs1DForOutWhenUnconnected=off
  x-distance [m] : Outport  Port=2  VectorParamsAs1DForOutWhenUnconnected=off
  y-distance [m] : Outport  Port=3  VectorParamsAs1DForOutWhenUnconnected=off
  lat acceleration [m/s^2] : Outport  Port=4  VectorParamsAs1DForOutWhenUnconnected=off
  lat velocity [m/s] : Outport  Port=5  VectorParamsAs1DForOutWhenUnconnected=off
  yaw rate [rad/s] : Outport  Port=6  VectorParamsAs1DForOutWhenUnconnected=off
  wires:
  __UniqueInportName__1__/1 -> long velocity [m/s]/1
  __UniqueInportName__2__/1 -> x-distance [m]/1
  __UniqueInportName__3__/1 -> y-distance [m]/1
  __UniqueInportName__4__/1 -> lat acceleration [m/s^2]/1
  __UniqueInportName__5__/1 -> lat velocity [m/s]/1
  __UniqueInportName__6__/1 -> yaw rate [rad/s]/1

== system MPC_HW2_Plant_Simulink/Subsystem1/Nonlinear Vehicle Model (9 DoF)1/__InputSSForSFun__ ==
  steering wheel angle [rad] : Inport
  target pre-maneuver speed [m/s] : Inport  Port=2
  Add yaw moment [Nm] : Inport  Port=3
  __UniqueOutportName__1__ : Outport
  __UniqueOutportName__2__ : Outport  Port=2
  __UniqueOutportName__3__ : Outport  Port=3
  wires:
  steering wheel angle [rad]/1 -> __UniqueOutportName__1__/1
  target pre-maneuver speed [m/s]/1 -> __UniqueOutportName__2__/1
  Add yaw moment [Nm]/1 -> __UniqueOutportName__3__/1

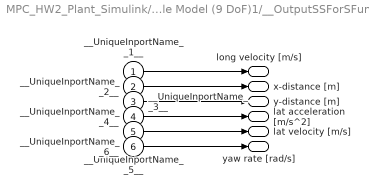
== system MPC_HW2_Plant_Simulink/Subsystem1/Nonlinear Vehicle Model (9 DoF)1/__OutputSSForSFun__ ==
  __UniqueInportName__1__ : Inport
  __UniqueInportName__2__ : Inport  Port=2
  __UniqueInportName__3__ : Inport  Port=3
  __UniqueInportName__4__ : Inport  Port=4
  __UniqueInportName__5__ : Inport  Port=5
  __UniqueInportName__6__ : Inport  Port=6
  long velocity [m/s] : Outport  VectorParamsAs1DForOutWhenUnconnected=off
  x-distance [m] : Outport  Port=2  VectorParamsAs1DForOutWhenUnconnected=off
  y-distance [m] : Outport  Port=3  VectorParamsAs1DForOutWhenUnconnected=off
  lat acceleration [m/s^2] : Outport  Port=4  VectorParamsAs1DForOutWhenUnconnected=off
  lat velocity [m/s] : Outport  Port=5  VectorParamsAs1DForOutWhenUnconnected=off
  yaw rate [rad/s] : Outport  Port=6  VectorParamsAs1DForOutWhenUnconnected=off
  wires:
  __UniqueInportName__1__/1 -> long velocity [m/s]/1
  __UniqueInportName__2__/1 -> x-distance [m]/1
  __UniqueInportName__3__/1 -> y-distance [m]/1
  __UniqueInportName__4__/1 -> lat acceleration [m/s^2]/1
  __UniqueInportName__5__/1 -> lat velocity [m/s]/1
  __UniqueInportName__6__/1 -> yaw rate [rad/s]/1

== system MPC_HW2_Plant_Simulink/Subsystem2/Nonlinear Vehicle Model (9 DoF)/__InputSSForSFun__ ==
  steering wheel angle [rad] : Inport
  target pre-maneuver speed [m/s] : Inport  Port=2
  Add yaw moment [Nm] : Inport  Port=3
  __UniqueOutportName__1__ : Outport
  __UniqueOutportName__2__ : Outport  Port=2
  __UniqueOutportName__3__ : Outport  Port=3
  wires:
  steering wheel angle [rad]/1 -> __UniqueOutportName__1__/1
  target pre-maneuver speed [m/s]/1 -> __UniqueOutportName__2__/1
  Add yaw moment [Nm]/1 -> __UniqueOutportName__3__/1

== system MPC_HW2_Plant_Simulink/Subsystem2/Nonlinear Vehicle Model (9 DoF)/__OutputSSForSFun__ ==
  __UniqueInportName__1__ : Inport
  __UniqueInportName__2__ : Inport  Port=2
  __UniqueInportName__3__ : Inport  Port=3
  __UniqueInportName__4__ : Inport  Port=4
  __UniqueInportName__5__ : Inport  Port=5
  __UniqueInportName__6__ : Inport  Port=6
  long velocity [m/s] : Outport  VectorParamsAs1DForOutWhenUnconnected=off
  x-distance [m] : Outport  Port=2  VectorParamsAs1DForOutWhenUnconnected=off
  y-distance [m] : Outport  Port=3  VectorParamsAs1DForOutWhenUnconnected=off
  lat acceleration [m/s^2] : Outport  Port=4  VectorParamsAs1DForOutWhenUnconnected=off
  lat velocity [m/s] : Outport  Port=5  VectorParamsAs1DForOutWhenUnconnected=off
  yaw rate [rad/s] : Outport  Port=6  VectorParamsAs1DForOutWhenUnconnected=off
  wires:
  __UniqueInportName__1__/1 -> long velocity [m/s]/1
  __UniqueInportName__2__/1 -> x-distance [m]/1
  __UniqueInportName__3__/1 -> y-distance [m]/1
  __UniqueInportName__4__/1 -> lat acceleration [m/s^2]/1
  __UniqueInportName__5__/1 -> lat velocity [m/s]/1
  __UniqueInportName__6__/1 -> yaw rate [rad/s]/1

== matlab function MPC_HW2_Plant_Simulink/Subsystem2/Regerence Generator/MATLAB Function ==
  data: delta input; u input; yawr_ss output; par parameter
function yawr_ss = bicycle_model(delta,u,par)
%Parameters
L = par.L;
g = par.g;
m = par.mass;
K = par.Kus;

%Yaw rate response
yawr_ss = u*delta/(L+K*u^2/g);

== matlab function MPC_HW2_Plant_Simulink/Subsystem1/MPC Controller (automatically updated after new code generation)1/Shift reference ==
  data: y output; yN input; Np parameter
function y = shift_reference(yN,Np)

y=repmat([yN;0],Np,1)';

end

== matlab function MPC_HW2_Plant_Simulink/Subsystem2/MPC Controller (automatically updated after new code generation)/Shift reference ==
  data: y output; yN input; Np parameter
function y = shift_reference(yN,Np)

y=repmat([yN;0],Np,1)';

end

== matlab function MPC_HW2_Plant_Simulink/Subsystem1/MPC Controller (automatically updated after new code generation)1/Shift reference2 ==
  data: y output; yN input; Np parameter
function y = shift_reference(yN,Np)

y=repmat(yN,Np+1,1)';

end

== matlab function MPC_HW2_Plant_Simulink/Subsystem2/MPC Controller (automatically updated after new code generation)/Shift reference2 ==
  data: y output; yN input; Np parameter
function y = shift_reference(yN,Np)

y=repmat(yN,Np+1,1)';

end

== matlab function MPC_HW2_Plant_Simulink/Subsystem1/Regerence Generator1/MATLAB Function ==
  data: delta input; u input; yawr_ss output; par parameter
function yawr_ss = bicycle_model(delta,u,par)
%Parameters
L = par.L;
g = par.g;
m = par.mass;
K = par.Kus;

%Yaw rate response
yawr_ss = u*delta/(L+K*u^2/g);

== matlab function MPC_HW2_Plant_Simulink/Subsystem1/Regerence Generator1/MATLAB Function1 ==
  data: yawr_ss input; u input; yawr_sat output; par parameter
function yawr_sat = boundary_conditions(yawr_ss,u,par)
g = par.g;
mu = par.mu;

yawr_max = 0.85*mu*g/u;

if abs(yawr_ss) > abs(yawr_max)
    yawr_sat = sign(yawr_ss)*yawr_max;
else
    yawr_sat = yawr_ss;
end

== matlab function MPC_HW2_Plant_Simulink/Subsystem/MPC Controller (automatically updated after new code generation)2/Shift reference ==
  data: y output; yN input; Np parameter
function y = shift_reference(yN,Np)

y=repmat([yN;0],Np,1)';

end

== matlab function MPC_HW2_Plant_Simulink/Subsystem/Regerence Generator2/MATLAB Function ==
  data: delta input; u input; yawr_ss output; par parameter
function yawr_ss = bicycle_model(delta,u,par)
%Parameters
L = par.L;
g = par.g;
m = par.mass;
K = par.Kus;

%Yaw rate response
yawr_ss = u*delta/(L+K*u^2/g);

== matlab function MPC_HW2_Plant_Simulink/Subsystem2/Regerence Generator/MATLAB Function1 ==
  data: yawr_ss input; u input; yawr_sat output; par parameter
function yawr_sat = boundary_conditions(yawr_ss,u,par)
g = par.g;
mu = par.mu;

yawr_max = 0.85*mu*g/u;

if abs(yawr_ss) > abs(yawr_max)
    yawr_sat = sign(yawr_ss)*yawr_max;
else
    yawr_sat = yawr_ss;
end

== matlab function MPC_HW2_Plant_Simulink/Subsystem/Regerence Generator2/MATLAB Function1 ==
  data: yawr_ss input; u input; yawr_sat output; par parameter
function yawr_sat = boundary_conditions(yawr_ss,u,par)
g = par.g;
mu = par.mu;

yawr_max = 0.85*mu*g/u;

if abs(yawr_ss) > abs(yawr_max)
    yawr_sat = sign(yawr_ss)*yawr_max;
else
    yawr_sat = yawr_ss;
end
